simulink model "ejemplo0317_motorDC_simulink"  (R2025b)
settings: Solver=VariableStepAuto  StartTime=0.0  StopTime=3  RelTol=1e-3
values from neighbouring files (symbols this model uses):
  B = 0.003026    [ejemplo0317_motorDC.m]    (also in ejemplo0324_LGR.m = 0.02; ejemplo0505_intronyquist.m = 2 + 2j; ejemplo0519_compensadoratrasoRF.m = 7.67361489362; ejemplo0611_REE.m = [1/L)
  J = 0.00246    [ejemplo0317_motorDC.m]    (also in ejemplo0324_LGR.m = 0.00625)
  Ka = 0.25    [ejemplo0317_motorDC.m]
  Km = 0.25    [ejemplo0317_motorDC.m]
  L = 0.0047    [ejemplo0317_motorDC.m]    (also in ejemplo0611_REE.m = 3; ejemplo0618_Observabilidad_Controlabilidad.m = 3)
  R = 2.27    [ejemplo0317_motorDC.m]    (also in ejemplo0430_FaseNominima.m = 0.746; ejemplo0611_REE.m = 100; ejemplo0618_Observabilidad_Controlabilidad.m = 100)
settings Model: Creator=cjuar  LastModifiedBy=cjuar

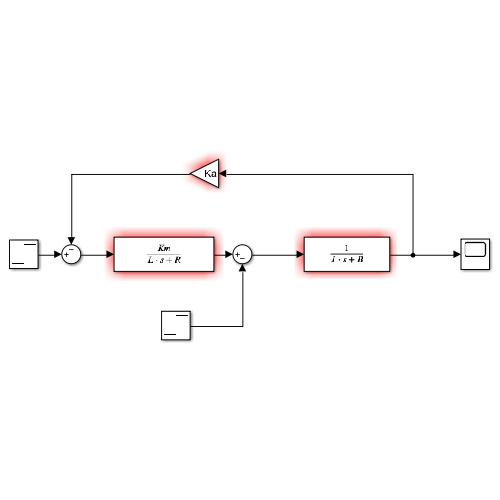
[thumbnail: Simulink's stored preview of the top-level diagram]
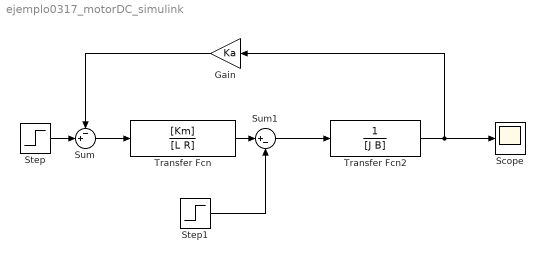
== system ejemplo0317_motorDC_simulink ==
  Gain : Gain  Gain=Ka
  Scope : Scope
  Step : Step  SampleTime=0
  Step1 : Step  After=0  SampleTime=0
  Sum : Sum  Inputs=-+|
  Sum1 : Sum  Inputs=|+-
  Transfer Fcn : TransferFcn  Numerator=[Km]  Denominator=[L R]
  Transfer Fcn2 : TransferFcn  Denominator=[J B]
  wires:
  Sum/1 -> Transfer Fcn/1
  Transfer Fcn/1 -> Sum1/1
  Sum1/1 -> Transfer Fcn2/1
  Transfer Fcn2/1 -> Scope/1, Gain/1
  Gain/1 -> Sum/1
  Step/1 -> Sum/2
  Step1/1 -> Sum1/2
